simulink model "gyro"  (R2023b)
settings: Solver=ode3  StartTime=t0  StopTime=tf  FixedStep=0.1  RelTol=1e-3
values from neighbouring files (symbols this model uses):
  I = [Ix, 0, 0; 0, Iy, 0; 0, 0, Iz]    [provaAttitudeCode.m]
  I_inv = inv(I)    [provaAttitudeCode.m]
undefined symbols (not defined in the file or in its folder): ARW, bias, M, omega_0, q_0, rot
libraries: matrix_library x2, simulink x1
settings Model: Creator=valen  LastModifiedBy=samue

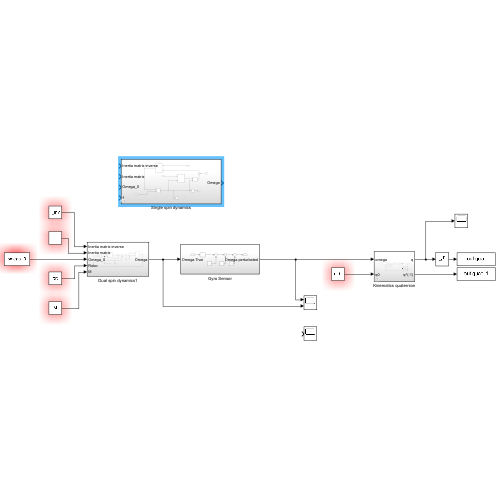
[thumbnail: Simulink's stored preview of the top-level diagram]
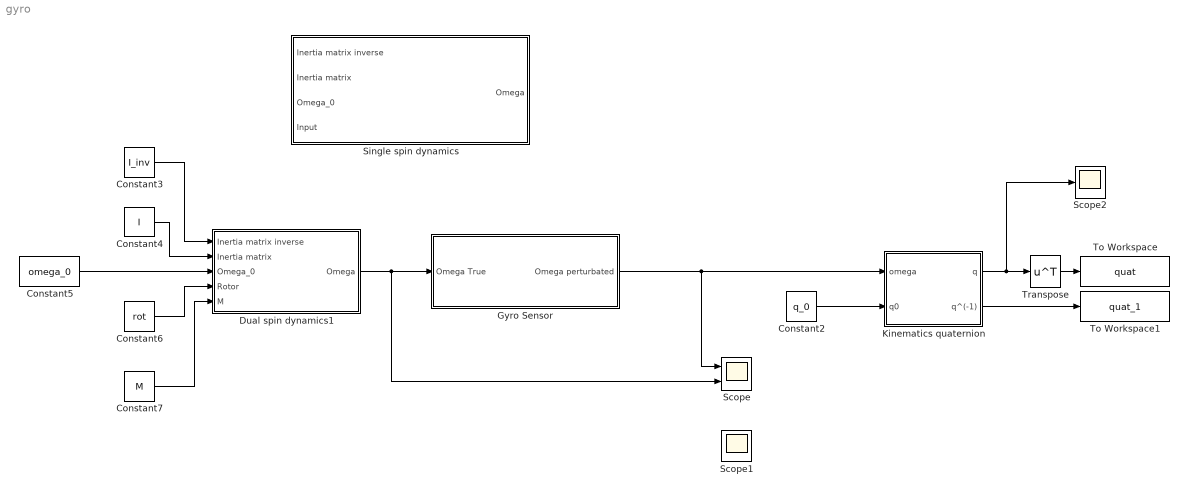
== system gyro ==
  Constant2 : Constant  Value=q_0  VectorParams1D=off
  Constant3 : Constant  Value=I_inv  VectorParams1D=off
  Constant4 : Constant  Value=I  VectorParams1D=off
  Constant5 : Constant  Value=omega_0  VectorParams1D=off
  Constant6 : Constant  Value=rot  VectorParams1D=off
  Constant7 : Constant  Value=M  VectorParams1D=off
  Dual spin dynamics1 : Subsystem
  Gyro Sensor : Subsystem
  Kinematics quaternion : Subsystem  AncestorBlock=LibrarySAD5/Kinematics quaternion
  Scope : Scope  NumInputPorts=2
  Scope1 : Scope
  Scope2 : Scope
  Single spin dynamics : Subsystem  AncestorBlock=My_library/Single spin dynamics
  To Workspace : ToWorkspace  VariableName=quat  SampleTime=-1
      settings: Save2DSignal=2-D array (concatenate along first dimension)
  To Workspace1 : ToWorkspace  VariableName=quat_1  SampleTime=-1
      settings: Save2DSignal=2-D array (concatenate along first dimension)
  Transpose : Math  Operator=transpose
  wires:
  Dual spin dynamics1/1(Omega) -> Scope/2, Gyro Sensor/1(Omega True)
  Constant2/1 -> Kinematics quaternion/2(q0)
  Constant3/1 -> Dual spin dynamics1/1(Inertia matrix inverse)
  Constant4/1 -> Dual spin dynamics1/2(Inertia matrix)
  Constant5/1 -> Dual spin dynamics1/3(Omega_0)
  Constant6/1 -> Dual spin dynamics1/4(Rotor)
  Constant7/1 -> Dual spin dynamics1/5(M)
  Kinematics quaternion/2(q^(-1)) -> To Workspace1/1
  Kinematics quaternion/1(q) -> Transpose/1, Scope2/1
  Transpose/1 -> To Workspace/1
  Gyro Sensor/1(Omega perturbated) -> Scope/1, Kinematics quaternion/1(omega)

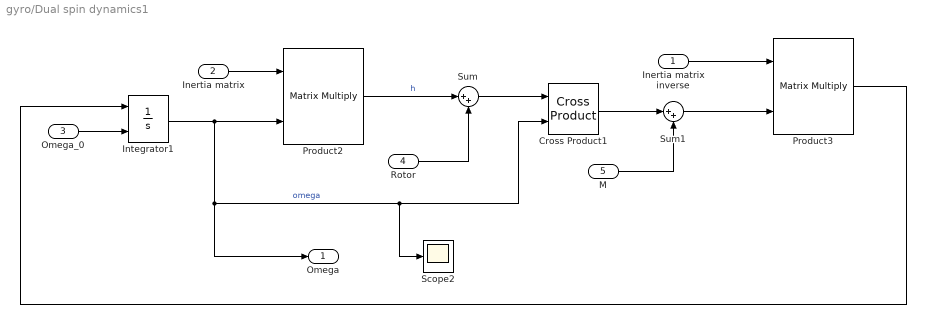
== system gyro/Dual spin dynamics1 ==
  Inertia matrix inverse : Inport
  Inertia matrix : Inport  Port=2
  Omega_0 : Inport  Port=3
  Rotor : Inport  Port=4
  M : Inport  Port=5
  Cross Product1 : matrix_library/Cross Product
  Integrator1 : Integrator  InitialConditionSource=external
  Product2 : Product  Multiplication=Matrix(*)
  Product3 : Product  Multiplication=Matrix(*)
  Scope2 : Scope
  Sum : Sum  Inputs=|++
  Sum1 : Sum  Inputs=|++
  Omega : Outport
  wires:
  M/1 -> Sum1/2
  Sum1/1 -> Product3/2
  Omega_0/1 -> Integrator1/2
  Product2/1 -> Sum/1  "h"
  Inertia matrix/1 -> Product2/1
  Product3/1 -> Integrator1/1
  Rotor/1 -> Sum/2
  Integrator1/1 -> Product2/2, Omega/1, Scope2/1, Cross Product1/2  "omega"
  Cross Product1/1 -> Sum1/1
  Inertia matrix inverse/1 -> Product3/1
  Sum/1 -> Cross Product1/1

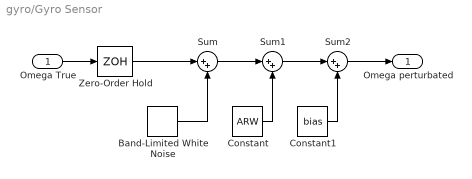
== system gyro/Gyro Sensor ==
  Omega True : Inport
  Band-Limited White Noise : simulink/Sources/Band-Limited White Noise  Cov=[0.00001]  Ts=0.1  seed=[23341]
  Constant : Constant  Value=ARW  VectorParams1D=off
  Constant1 : Constant  Value=bias  VectorParams1D=off
  Sum : Sum  Inputs=|++
  Sum1 : Sum  Inputs=|++
  Sum2 : Sum  Inputs=|++
  Zero-Order Hold : ZeroOrderHold  SampleTime=-1
  Omega perturbated : Outport
  wires:
  Zero-Order Hold/1 -> Sum/1
  Sum2/1 -> Omega perturbated/1
  Sum1/1 -> Sum2/1
  Sum/1 -> Sum1/1
  Omega True/1 -> Zero-Order Hold/1
  Constant1/1 -> Sum2/2
  Band-Limited White Noise/1 -> Sum/2
  Constant/1 -> Sum1/2

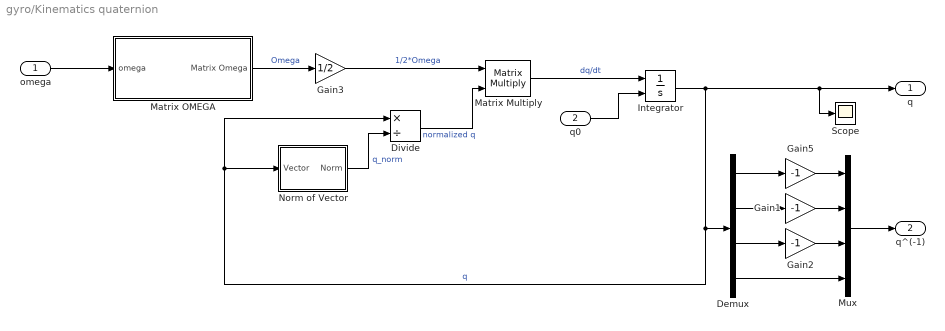
== system gyro/Kinematics quaternion ==
  omega : Inport
  q0 : Inport  Port=2
  Demux : Demux
  Divide : Product  Inputs=*/
  Gain1 : Gain  Gain=-1
  Gain2 : Gain  Gain=-1
  Gain3 : Gain  Gain=1/2
  Gain5 : Gain  Gain=-1
  Integrator : Integrator  InitialConditionSource=external
  Matrix Multiply : Product  Multiplication=Matrix(*)
  Matrix OMEGA : Subsystem
  Mux : Mux
  Norm of Vector : Subsystem
  Scope : Scope
  q : Outport
  q^(-1) : Outport  Port=2
  wires:
  Gain5/1 -> Mux/1
  Demux/1 -> Gain5/1
  Divide/1 -> Matrix Multiply/2  "normalized q"
  Norm of Vector/1(Norm) -> Divide/2  "q_norm"
  Mux/1 -> q^(-1)/1
  Demux/4 -> Mux/4
  Gain2/1 -> Mux/3
  Gain1/1 -> Mux/2
  Demux/3 -> Gain2/1
  Demux/2 -> Gain1/1
  q0/1 -> Integrator/2
  Matrix OMEGA/1(Matrix Omega) -> Gain3/1  "Omega"
  Integrator/1 -> Demux/1, Divide/1, Norm of Vector/1(Vector), q/1, Scope/1  "q"
  omega/1 -> Matrix OMEGA/1(omega)
  Matrix Multiply/1 -> Integrator/1  "dq/dt"
  Gain3/1 -> Matrix Multiply/1  "1/2*Omega"

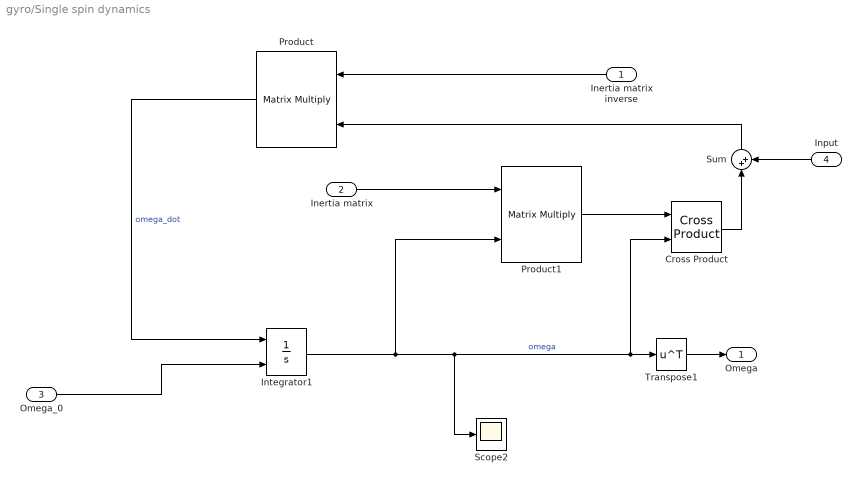
== system gyro/Single spin dynamics ==
  Inertia matrix inverse : Inport
  Inertia matrix : Inport  Port=2
  Omega_0 : Inport  Port=3
  Input : Inport  Port=4
  Cross Product : matrix_library/Cross Product
  Integrator1 : Integrator  InitialConditionSource=external
  Product : Product  Multiplication=Matrix(*)
  Product1 : Product  Multiplication=Matrix(*)
  Scope2 : Scope
  Sum : Sum  Inputs=|++
  Transpose1 : Math  Operator=transpose
  Omega : Outport
  wires:
  Transpose1/1 -> Omega/1
  Inertia matrix inverse/1 -> Product/1
  Integrator1/1 -> Product1/2, Transpose1/1, Cross Product/2, Scope2/1  "omega"
  Product/1 -> Integrator1/1  "omega_dot"
  Omega_0/1 -> Integrator1/2
  Product1/1 -> Cross Product/1
  Inertia matrix/1 -> Product1/1
  Cross Product/1 -> Sum/1
  Sum/1 -> Product/2
  Input/1 -> Sum/2

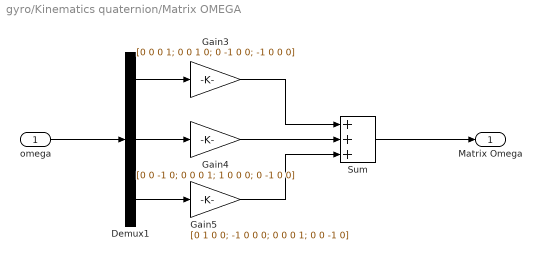
== system gyro/Kinematics quaternion/Matrix OMEGA ==
  omega : Inport
  Demux1 : Demux  Outputs=3
  Gain3 : Gain  Gain=[0 0 0 1; 0 0 1 0; 0 -1 0 0; -1 0 0 0]
  Gain4 : Gain  Gain=[0 0 -1 0; 0 0 0 1; 1 0 0 0; 0 -1 0 0]
  Gain5 : Gain  Gain=[0 1 0 0; -1 0 0 0; 0 0 0 1; 0 0 -1 0]
  Sum : Sum  Inputs=+++
  Matrix Omega : Outport
  wires:
  Gain5/1 -> Sum/3
  Gain4/1 -> Sum/2
  Gain3/1 -> Sum/1
  Demux1/1 -> Gain3/1
  omega/1 -> Demux1/1
  Demux1/2 -> Gain4/1
  Demux1/3 -> Gain5/1
  Sum/1 -> Matrix Omega/1

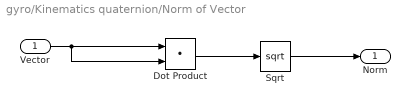
== system gyro/Kinematics quaternion/Norm of Vector ==
  Vector : Inport
  Dot Product : DotProduct  OutDataTypeStr=Inherit: Inherit via internal rule
  Sqrt : Sqrt
  Norm : Outport
  wires:
  Dot Product/1 -> Sqrt/1
  Vector/1 -> Dot Product/2, Dot Product/1
  Sqrt/1 -> Norm/1
